simulink model "P4_Combined_Electric_Vehicle"  (R2023b)
settings: Solver=VariableStepAuto  StartTime=0.0  StopTime=10.0  RelTol=1e-3
undefined symbols (not defined in the file or in its folder): batData, carData, motorData
settings Model: Creator=chris  LastModifiedBy=chris

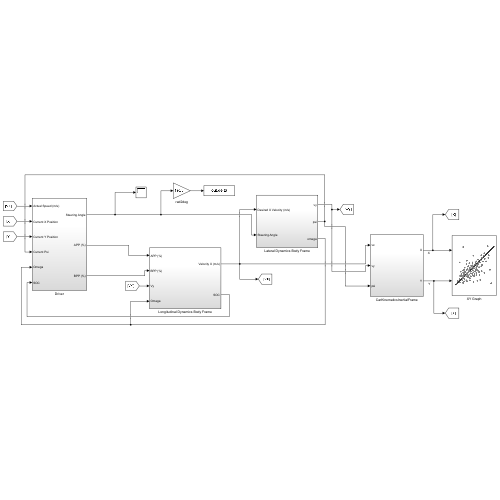
[thumbnail: Simulink's stored preview of the top-level diagram]
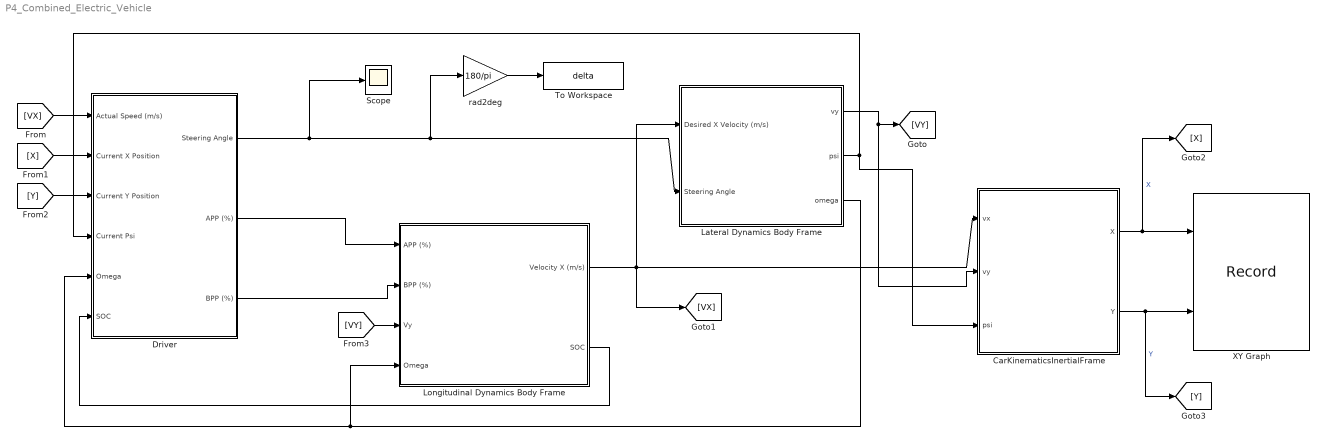
== system P4_Combined_Electric_Vehicle ==
  CarKinematicsInertialFrame : Subsystem
  Driver : Subsystem
  Lateral Dynamics Body Frame : Subsystem
  Longitudinal Dynamics Body Frame : Subsystem
  Scope : Scope
  To Workspace : ToWorkspace  VariableName=delta  SaveFormat=Timeseries  SampleTime=-1
  XY Graph : Record  FileSettingsInternal="{\"entries\":[{\"content\":{\"excelSettings\":{\"content\":{},\"type\":\"Streamout.ExcelSettings\"}},\"type\":\"Streamout.FileSettingStorage\",\"uuid\":\"\"}],\"packageUris\":[\"http:\\/\\/schema.mathworks.com\\/mf0\\/streamout_blocks\\/R2020a\"],\"version\":\"1.0\"}"  Layout=[1 1]  SignalsInternal="{\"entries\":[{\"content\":{\"signals\":[{\"content\":{\"blockPath\":[],\"dimensions\":[1],\"domain\":\"\",\"lineColor\":\"#a2142f\",\"plots\":[1],\"port\":1,\"signalID\":70,\"signalName\":\"XY Graph:1\"},\"type\":\"RecordBlkView.Signal\",\"uuid\":\"\"},{\"content\":{\"blockPath\":[],\"dimensions\":[1],\"domain\":\"\",\"lineColor\":\"#139fff\",\"plots\":[1],\"port\":2,\"signalID\":73,\"signalName\":\"XY Graph:2\"},\"type\":\"RecordBlkView.Signal\",\"uuid\":\"\"}]},\"type\":\"RecordBlkView.InputSignals\",\"uuid\":\"\"}],\"packageUris\":[\"http:\\/\\/schema.mathworks.com\\/mf0\\/streamout_blocks\\/R2020a\"],\"version\":\"1.0\"}"  VisualizationBindings="{\"xyplotplugin\":{\"info\":[{\"series\":[{\"bindingParametersList\":[{\"parameter\":\"X-Axis\",\"signalID\":70,\"signalName\":\"XY Graph:1\"},{\"parameter\":\"Y-Axis\",\"signalID\":73,\"signalName\":\"XY Graph:2\"}],\"seriesID\":10699}],\"subplotID\":1}]}}"  CompatibilityTag=XY
  rad2deg : Gain  Gain=180/pi
  wires:
  [VX] -> Driver/1(Actual Speed (m/s))
  [X] -> Driver/2(Current X Position)
  [Y] -> Driver/3(Current Y Position)
  Driver/2(APP (%)) -> Longitudinal Dynamics Body Frame/1(APP (%))
  Driver/3(BPP (%)) -> Longitudinal Dynamics Body Frame/2(BPP (%))
  [VY] -> Longitudinal Dynamics Body Frame/3(Vy)
  Driver/1(Steering Angle) -> rad2deg/1, Lateral Dynamics Body Frame/2(Steering Angle), Scope/1
  Longitudinal Dynamics Body Frame/1(Velocity X (m/s)) -> Lateral Dynamics Body Frame/1(Desired X Velocity (m/s)), CarKinematicsInertialFrame/1(vx), [VX]
  Longitudinal Dynamics Body Frame/2(SOC) -> Driver/6(SOC)
  rad2deg/1 -> To Workspace/1
  CarKinematicsInertialFrame/1(X) -> XY Graph/1, [X]  "X"
  CarKinematicsInertialFrame/2(Y) -> XY Graph/2, [Y]  "Y"
  Lateral Dynamics Body Frame/1(vy) -> CarKinematicsInertialFrame/2(vy), [VY]
  Lateral Dynamics Body Frame/2(psi) -> CarKinematicsInertialFrame/3(psi), Driver/4(Current Psi)
  Lateral Dynamics Body Frame/3(omega) -> Longitudinal Dynamics Body Frame/4(Omega), Driver/5(Omega)

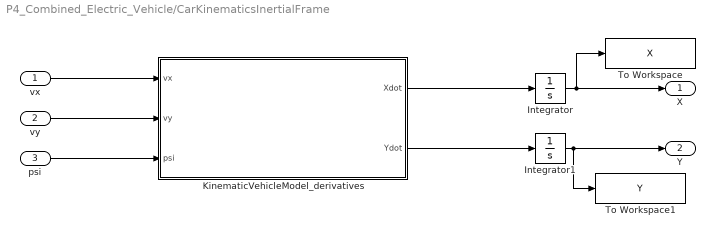
== system P4_Combined_Electric_Vehicle/CarKinematicsInertialFrame ==
  vx : Inport
  vy : Inport  Port=2
  psi : Inport  Port=3
  Integrator : Integrator  InitialCondition=carData.init.X0
  Integrator1 : Integrator  InitialCondition=carData.init.Y0
  KinematicVehicleModel_derivatives : MATLAB Function  TreatAsAtomicUnit=on  mask{obj=carData}
      mask prompts: obj "obj structure"
  To Workspace : ToWorkspace  VariableName=X  SaveFormat=Timeseries  SampleTime=-1
  To Workspace1 : ToWorkspace  VariableName=Y  SaveFormat=Timeseries  SampleTime=-1
  X : Outport
  Y : Outport  Port=2
  wires:
  KinematicVehicleModel_derivatives/1(Xdot) -> Integrator/1
  Integrator/1 -> X/1, To Workspace/1
  psi/1 -> KinematicVehicleModel_derivatives/3(psi)
  Integrator1/1 -> Y/1, To Workspace1/1
  vx/1 -> KinematicVehicleModel_derivatives/1(vx)
  vy/1 -> KinematicVehicleModel_derivatives/2(vy)
  KinematicVehicleModel_derivatives/2(Ydot) -> Integrator1/1

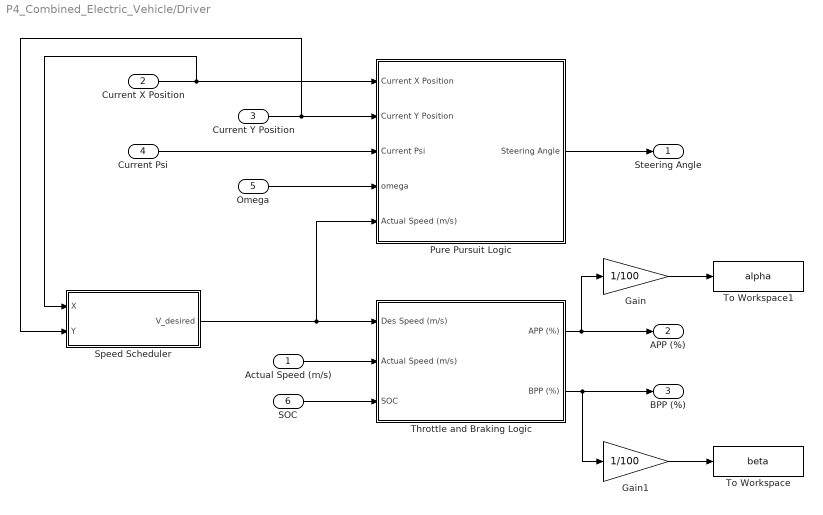
== system P4_Combined_Electric_Vehicle/Driver ==
  Actual Speed (m/s) : Inport
  Current X Position : Inport  Port=2
  Current Y Position : Inport  Port=3
  Current Psi : Inport  Port=4
  Omega : Inport  Port=5
  SOC : Inport  Port=6
  Gain : Gain  Gain=1/100
  Gain1 : Gain  Gain=1/100
  Pure Pursuit Logic : Subsystem
  Speed Scheduler : MATLAB Function  TreatAsAtomicUnit=on
  Throttle and Braking Logic : Subsystem
  To Workspace : ToWorkspace  VariableName=beta  SaveFormat=Timeseries  SampleTime=-1
  To Workspace1 : ToWorkspace  VariableName=alpha  SaveFormat=Timeseries  SampleTime=-1
  Steering Angle : Outport
  APP (%) : Outport  Port=2
  BPP (%) : Outport  Port=3
  wires:
  Actual Speed (m/s)/1 -> Throttle and Braking Logic/2(Actual Speed (m/s))
  SOC/1 -> Throttle and Braking Logic/3(SOC)
  Speed Scheduler/1(V_desired) -> Pure Pursuit Logic/5(Actual Speed (m/s)), Throttle and Braking Logic/1(Des Speed (m/s))
  Omega/1 -> Pure Pursuit Logic/4(omega)
  Current Y Position/1 -> Speed Scheduler/2(Y), Pure Pursuit Logic/2(Current Y Position)
  Current X Position/1 -> Speed Scheduler/1(X), Pure Pursuit Logic/1(Current X Position)
  Current Psi/1 -> Pure Pursuit Logic/3(Current Psi)
  Pure Pursuit Logic/1(Steering Angle) -> Steering Angle/1
  Throttle and Braking Logic/1(APP (%)) -> Gain/1, APP (%)/1
  Throttle and Braking Logic/2(BPP (%)) -> Gain1/1, BPP (%)/1
  Gain1/1 -> To Workspace/1
  Gain/1 -> To Workspace1/1

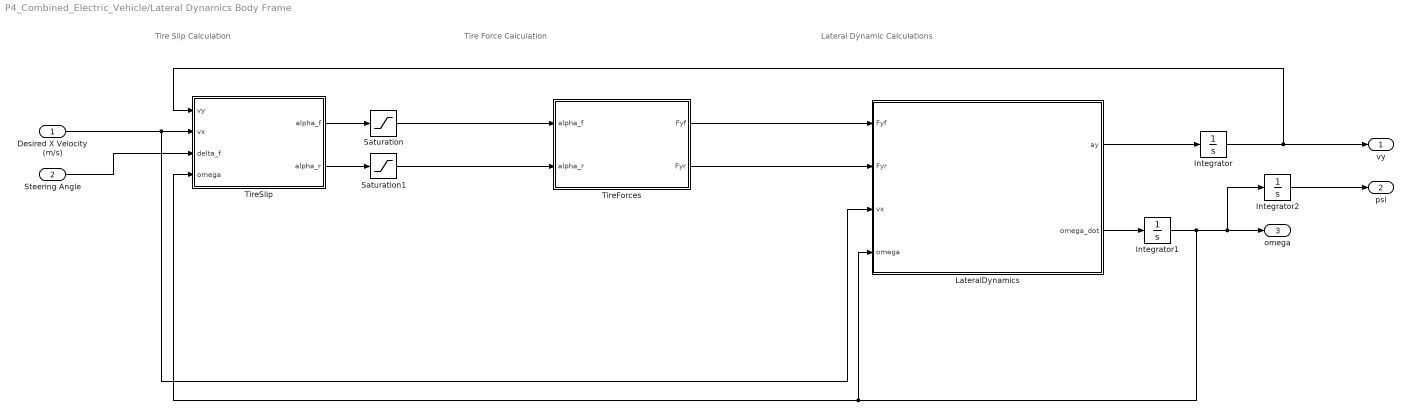
== system P4_Combined_Electric_Vehicle/Lateral Dynamics Body Frame ==
  note: Lateral Dynamic Calculations
  note: Tire Slip Calculation
  note: Tire Force Calculation
  Desired X Velocity (m/s) : Inport
  Steering Angle : Inport  Port=2
  Integrator : Integrator  InitialCondition=carData.init.vy0
  Integrator1 : Integrator  InitialCondition=carData.init.omega0
  Integrator2 : Integrator  InitialCondition=carData.init.psi0
  LateralDynamics : MATLAB Function  TreatAsAtomicUnit=on  mask{obj=carData}
      mask prompts: obj "obj structure"
  Saturation : Saturate  UpperLimit=carData.maxAlpha  LowerLimit=-carData.maxAlpha
  Saturation1 : Saturate  UpperLimit=carData.maxAlpha  LowerLimit=-carData.maxAlpha
  TireForces : MATLAB Function  TreatAsAtomicUnit=on  mask{obj=carData}
      mask prompts: obj "obj structure"
  TireSlip : MATLAB Function  TreatAsAtomicUnit=on  mask{obj=carData}
      mask prompts: obj "obj structure"
  vy : Outport
  psi : Outport  Port=2
  omega : Outport  Port=3
  wires:
  Integrator2/1 -> psi/1
  Steering Angle/1 -> TireSlip/3(delta_f)
  Desired X Velocity (m/s)/1 -> TireSlip/2(vx), LateralDynamics/3(vx)
  Saturation1/1 -> TireForces/2(alpha_r)
  TireForces/2(Fyr) -> LateralDynamics/2(Fyr)
  Saturation/1 -> TireForces/1(alpha_f)
  Integrator1/1 -> Integrator2/1, omega/1, LateralDynamics/4(omega), TireSlip/4(omega)
  Integrator/1 -> vy/1, TireSlip/1(vy)
  TireSlip/2(alpha_r) -> Saturation1/1
  LateralDynamics/2(omega_dot) -> Integrator1/1
  TireForces/1(Fyf) -> LateralDynamics/1(Fyf)
  TireSlip/1(alpha_f) -> Saturation/1
  LateralDynamics/1(ay) -> Integrator/1

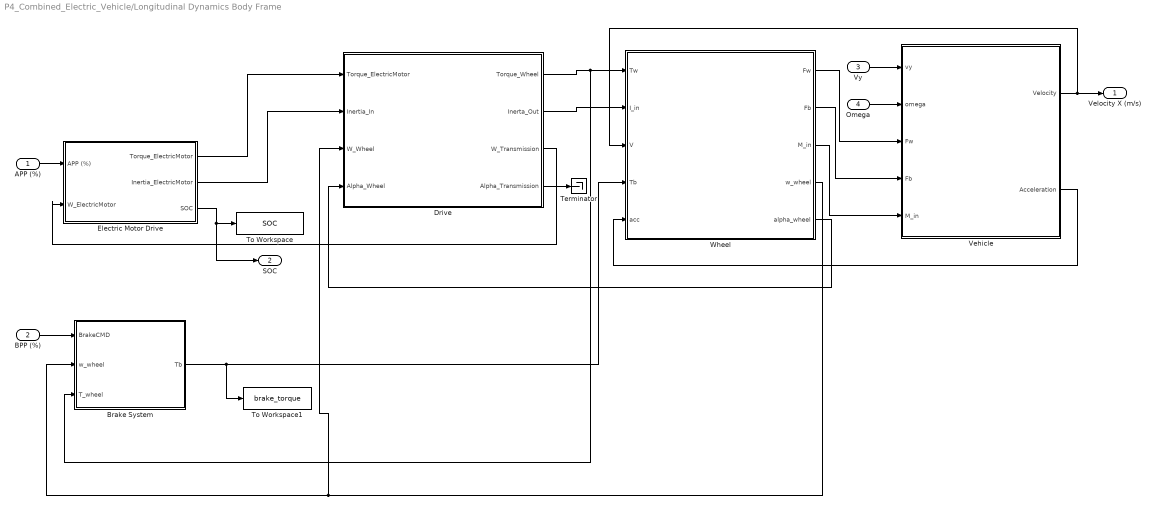
== system P4_Combined_Electric_Vehicle/Longitudinal Dynamics Body Frame ==
  APP (%) : Inport
  BPP (%) : Inport  Port=2
  Vy : Inport  Port=3
  Omega : Inport  Port=4
  Brake System : Subsystem
  Drive : Subsystem
  Electric Motor Drive : Subsystem
  Terminator : Terminator
  To Workspace : ToWorkspace  VariableName=SOC  SaveFormat=Timeseries  SampleTime=-1
  To Workspace1 : ToWorkspace  VariableName=brake_torque  SaveFormat=Timeseries  SampleTime=-1
  Vehicle : Subsystem
  Wheel : Subsystem
  Velocity X (m/s) : Outport
  SOC : Outport  Port=2
  wires:
  Vy/1 -> Vehicle/1(vy)
  Omega/1 -> Vehicle/2(omega)
  APP (%)/1 -> Electric Motor Drive/1(APP (%))
  Electric Motor Drive/3(SOC) -> To Workspace/1, SOC/1
  BPP (%)/1 -> Brake System/1("BrakeCMD ")
  Drive/4(Alpha_Transmission) -> Terminator/1
  Electric Motor Drive/1(Torque_ElectricMotor) -> Drive/1(Torque_ElectricMotor)
  Electric Motor Drive/2(Inertia_ElectricMotor) -> Drive/2(Inertia_In)
  Wheel/3(M_in) -> Vehicle/5("M_in ")
  Wheel/2(Fb) -> Vehicle/4(Fb)
  Wheel/1(Fw) -> Vehicle/3("Fw ")
  Vehicle/2(Acceleration) -> Wheel/5(acc)
  Vehicle/1("Velocity ") -> Wheel/3(V), Velocity X (m/s)/1
  Drive/1(Torque_Wheel) -> Wheel/1(Tw), Brake System/3(T_wheel)
  Drive/2(Inerta_Out) -> Wheel/2(I_in)
  Brake System/1(Tb) -> To Workspace1/1, Wheel/4(Tb)
  Drive/3(W_Transmission) -> Electric Motor Drive/2(W_ElectricMotor)
  Wheel/5(alpha_wheel) -> Drive/4(Alpha_Wheel)
  Wheel/4(w_wheel) -> Drive/3(W_Wheel), Brake System/2("w_wheel ")

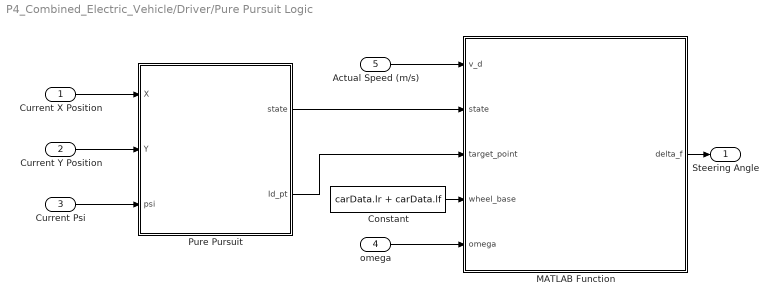
== system P4_Combined_Electric_Vehicle/Driver/Pure Pursuit Logic ==
  Current X Position : Inport
  Current Y Position : Inport  Port=2
  Current Psi : Inport  Port=3
  omega : Inport  Port=4
  Actual Speed (m/s) : Inport  Port=5
  Constant : Constant  Value=carData.lr + carData.lf
  MATLAB Function : MATLAB Function  TreatAsAtomicUnit=on
  Pure Pursuit : MATLAB Function  TreatAsAtomicUnit=on
  Steering Angle : Outport
  wires:
  Current X Position/1 -> Pure Pursuit/1(X)
  Current Y Position/1 -> Pure Pursuit/2(Y)
  Current Psi/1 -> Pure Pursuit/3(psi)
  Actual Speed (m/s)/1 -> MATLAB Function/1(v_d)
  Pure Pursuit/1(state) -> MATLAB Function/2(state)
  omega/1 -> MATLAB Function/5(omega)
  Pure Pursuit/2(Id_pt) -> MATLAB Function/3(target_point)
  MATLAB Function/1(delta_f) -> Steering Angle/1
  Constant/1 -> MATLAB Function/4(wheel_base)

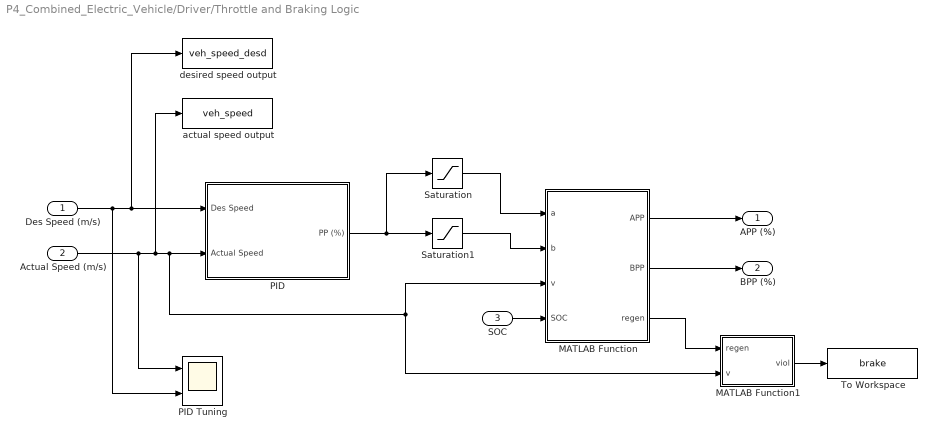
== system P4_Combined_Electric_Vehicle/Driver/Throttle and Braking Logic ==
  Des Speed (m/s) : Inport
  Actual Speed (m/s) : Inport  Port=2
  SOC : Inport  Port=3
  MATLAB Function : MATLAB Function  TreatAsAtomicUnit=on
  MATLAB Function1 : MATLAB Function  TreatAsAtomicUnit=on
  PID : Subsystem
  PID Tuning : Scope  NumInputPorts=2
  Saturation : Saturate  UpperLimit=1  LowerLimit=0
  Saturation1 : Saturate  UpperLimit=0  LowerLimit=-1
  To Workspace : ToWorkspace  VariableName=brake  SaveFormat=Timeseries  SampleTime=-1
  actual speed output : ToWorkspace  VariableName=veh_speed  SaveFormat=Timeseries  SampleTime=-1
  desired speed output : ToWorkspace  VariableName=veh_speed_desd  SaveFormat=Timeseries  SampleTime=-1
  APP (%) : Outport
  BPP (%) : Outport  Port=2
  wires:
  Des Speed (m/s)/1 -> desired speed output/1, PID/1(Des Speed), PID Tuning/2
  Actual Speed (m/s)/1 -> PID Tuning/1, actual speed output/1, MATLAB Function1/2(v), MATLAB Function/3(v), PID/2(Actual Speed)
  SOC/1 -> MATLAB Function/4(SOC)
  MATLAB Function/1(APP) -> APP (%)/1
  MATLAB Function/2(BPP) -> BPP (%)/1
  PID/1(PP (%)) -> Saturation1/1, Saturation/1
  Saturation1/1 -> MATLAB Function/2(b)
  Saturation/1 -> MATLAB Function/1(a)
  MATLAB Function/3(regen) -> MATLAB Function1/1(regen)
  MATLAB Function1/1(viol) -> To Workspace/1

== system P4_Combined_Electric_Vehicle/Longitudinal Dynamics Body Frame/Brake System ==
  "BrakeCMD " : Inport
  "w_wheel " : Inport  Port=2
  T_wheel : Inport  Port=3
  Gain1 : Gain  Gain=10000
  MATLAB Function : MATLAB Function  TreatAsAtomicUnit=on
  Tb : Outport  VectorParamsAs1DForOutWhenUnconnected=off
  wires:
  "BrakeCMD "/1 -> Gain1/1
  T_wheel/1 -> MATLAB Function/3(T_wheel)
  "w_wheel "/1 -> MATLAB Function/2(v)
  Gain1/1 -> MATLAB Function/1(Tbcap)
  MATLAB Function/1(Tb) -> Tb/1

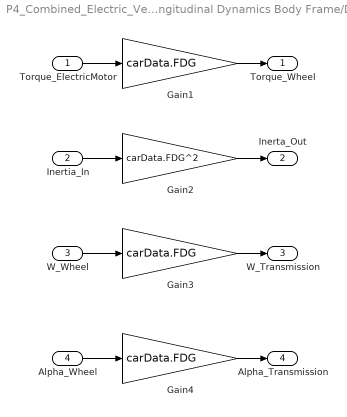
== system P4_Combined_Electric_Vehicle/Longitudinal Dynamics Body Frame/Drive ==
  Torque_ElectricMotor : Inport
  Inertia_In : Inport  Port=2
  W_Wheel : Inport  Port=3
  Alpha_Wheel : Inport  Port=4
  Gain1 : Gain  Gain=carData.FDG
  Gain2 : Gain  Gain=carData.FDG^2
  Gain3 : Gain  Gain=carData.FDG
  Gain4 : Gain  Gain=carData.FDG
  Torque_Wheel : Outport
  Inerta_Out : Outport  Port=2
  W_Transmission : Outport  Port=3
  Alpha_Transmission : Outport  Port=4
  wires:
  Inertia_In/1 -> Gain2/1
  Torque_ElectricMotor/1 -> Gain1/1
  Gain4/1 -> Alpha_Transmission/1
  Gain2/1 -> Inerta_Out/1
  Gain1/1 -> Torque_Wheel/1
  W_Wheel/1 -> Gain3/1
  Gain3/1 -> W_Transmission/1
  Alpha_Wheel/1 -> Gain4/1

== system P4_Combined_Electric_Vehicle/Longitudinal Dynamics Body Frame/Electric Motor Drive ==
  APP (%) : Inport
  W_ElectricMotor : Inport  Port=2
  Battery : Subsystem
  Electric Motor : Subsystem
  Torque_ElectricMotor : Outport
  Inertia_ElectricMotor : Outport  Port=2
  SOC : Outport  Port=3
  wires:
  Electric Motor/3(Inertia_ElectricMotor) -> Inertia_ElectricMotor/1
  Electric Motor/2(Torque_ElectricMotor) -> Torque_ElectricMotor/1
  Battery/2(SOC) -> SOC/1
  Electric Motor/1(I_bat) -> Battery/1(I_battery)
  APP (%)/1 -> Electric Motor/2(APP (%))
  W_ElectricMotor/1 -> Electric Motor/3(W_ElectricMotor)
  Battery/1(V_bat) -> Electric Motor/1(Bat Voltage)

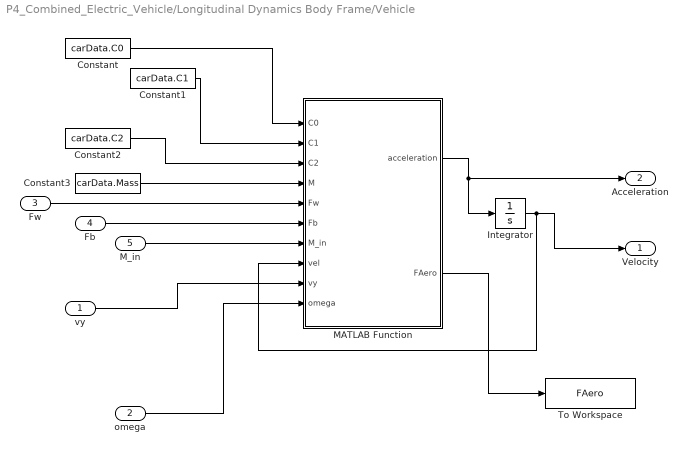
== system P4_Combined_Electric_Vehicle/Longitudinal Dynamics Body Frame/Vehicle ==
  vy : Inport
  omega : Inport  Port=2
  "Fw " : Inport  Port=3
  Fb : Inport  Port=4
  "M_in " : Inport  Port=5
  Constant : Constant  Value=carData.C0
  Constant1 : Constant  Value=carData.C1
  Constant2 : Constant  Value=carData.C2
  Constant3 : Constant  Value=carData.Mass
  Integrator : Integrator  LimitOutput=on  LowerSaturationLimit=0
  MATLAB Function : MATLAB Function  TreatAsAtomicUnit=on
  To Workspace : ToWorkspace  VariableName=FAero  SaveFormat=Timeseries  SampleTime=-1
  "Velocity " : Outport  VectorParamsAs1DForOutWhenUnconnected=off
  Acceleration : Outport  Port=2
  wires:
  "M_in "/1 -> MATLAB Function/7(M_in)
  Constant3/1 -> MATLAB Function/4(M)
  "Fw "/1 -> MATLAB Function/5(Fw)
  Constant/1 -> MATLAB Function/1(C0)
  Constant2/1 -> MATLAB Function/3(C2)
  Fb/1 -> MATLAB Function/6(Fb)
  Integrator/1 -> "Velocity "/1, MATLAB Function/8(vel)
  MATLAB Function/1(acceleration) -> Integrator/1, Acceleration/1
  Constant1/1 -> MATLAB Function/2(C1)
  vy/1 -> MATLAB Function/9(vy)
  omega/1 -> MATLAB Function/10(omega)
  MATLAB Function/2(FAero) -> To Workspace/1

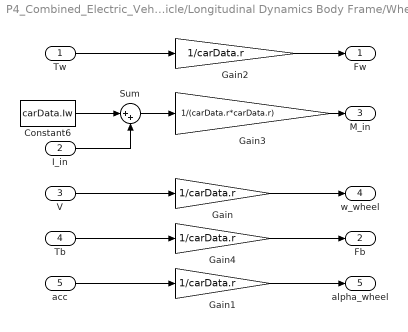
== system P4_Combined_Electric_Vehicle/Longitudinal Dynamics Body Frame/Wheel ==
  Tw : Inport
  I_in : Inport  Port=2
  V : Inport  Port=3
  Tb : Inport  Port=4
  acc : Inport  Port=5
  Constant6 : Constant  Value=carData.Iw
  Gain{,1..2,4} (4 alike) : Gain  Gain=1/carData.r
  Gain3 : Gain  Gain=1/(carData.r*carData.r)
  Sum : Sum  Inputs=|++
  Fw : Outport
  Fb : Outport  Port=2
  M_in : Outport  Port=3
  w_wheel : Outport  Port=4
  alpha_wheel : Outport  Port=5
  wires:
  acc/1 -> Gain1/1
  Gain1/1 -> alpha_wheel/1
  Constant6/1 -> Sum/1
  Gain3/1 -> M_in/1
  Sum/1 -> Gain3/1
  Gain4/1 -> Fb/1
  I_in/1 -> Sum/2
  V/1 -> Gain/1
  Tw/1 -> Gain2/1
  Gain/1 -> w_wheel/1
  Gain2/1 -> Fw/1
  Tb/1 -> Gain4/1

== system P4_Combined_Electric_Vehicle/Driver/Throttle and Braking Logic/PID ==
  Des Speed : Inport
  Actual Speed : Inport  Port=2
  PP (%) : Outport
  wires:
  Des Speed/1 -> PP (%)/1

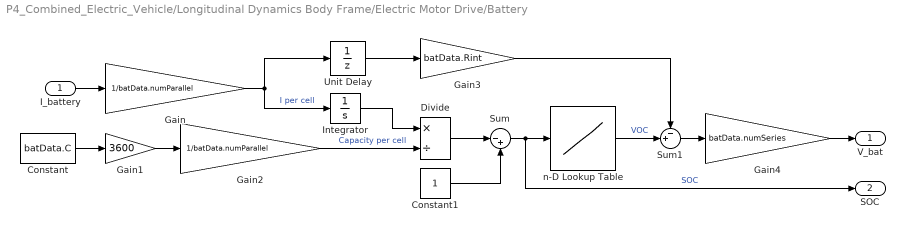
== system P4_Combined_Electric_Vehicle/Longitudinal Dynamics Body Frame/Electric Motor Drive/Battery ==
  I_battery : Inport
  Constant : Constant  Value=batData.C
  Constant1 : Constant
  Divide : Product  Inputs=*/
  Gain : Gain  Gain=1/batData.numParallel
  Gain1 : Gain  Gain=3600
  Gain2 : Gain  Gain=1/batData.numParallel
  Gain3 : Gain  Gain=batData.Rint
  Gain4 : Gain  Gain=batData.numSeries
  Integrator : Integrator
  Sum : Sum  Inputs=|-+
  Sum1 : Sum  Inputs=-+|
  Unit Delay : UnitDelay  SampleTime=-1  HasFrameUpgradeWarning=on
  n-D Lookup Table : Lookup_n-D  NumberOfTableDimensions=1  BreakpointsForDimension1=batData.SOC  BreakpointsForDimension3=[5, 7]  Table=batData.OCV  InternalRulePriority=Speed  RndMeth=Simplest
  V_bat : Outport
  SOC : Outport  Port=2
  wires:
  I_battery/1 -> Gain/1
  Gain/1 -> Unit Delay/1, Integrator/1  "I per cell"
  Constant/1 -> Gain1/1
  Gain1/1 -> Gain2/1
  Gain2/1 -> Divide/2  "Capacity per cell"
  Integrator/1 -> Divide/1
  Divide/1 -> Sum/1
  Constant1/1 -> Sum/2
  Sum/1 -> SOC/1, n-D Lookup Table/1  "SOC"
  Unit Delay/1 -> Gain3/1
  n-D Lookup Table/1 -> Sum1/2  "VOC"
  Gain3/1 -> Sum1/1
  Gain4/1 -> V_bat/1
  Sum1/1 -> Gain4/1

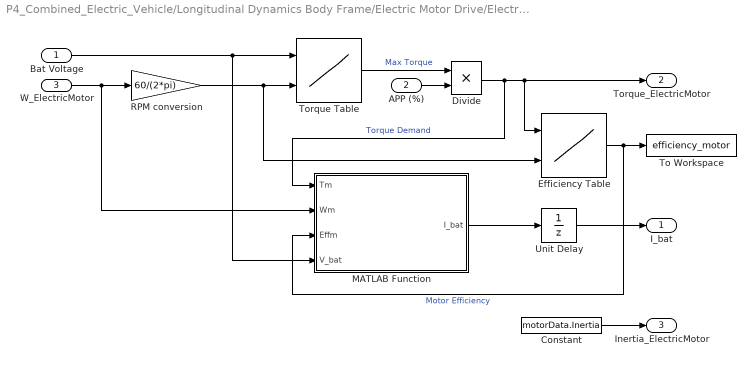
== system P4_Combined_Electric_Vehicle/Longitudinal Dynamics Body Frame/Electric Motor Drive/Electric Motor ==
  Bat Voltage : Inport
  APP (%) : Inport  Port=2
  W_ElectricMotor : Inport  Port=3
  Constant : Constant  Value=motorData.Inertia
  Divide : Product  Inputs=**
  Efficiency Table : Lookup_n-D  BreakpointsForDimension1=motorData.eta_torque  BreakpointsForDimension2=motorData.eta_speed  BreakpointsForDimension3=[5, 7]  Table=motorData.eta_val  ExtrapMethod=Clip  UseLastTableValue=on  InternalRulePriority=Speed  RndMeth=Simplest
      settings: InputPortMap=u0,u1
  MATLAB Function : MATLAB Function  TreatAsAtomicUnit=on
  RPM conversion : Gain  Gain=60/(2*pi)
  To Workspace : ToWorkspace  VariableName=efficiency_motor  SaveFormat=Timeseries  SampleTime=-1
  Torque Table : Lookup_n-D  BreakpointsForDimension1=motorData.vbus  BreakpointsForDimension2=motorData.rpm  BreakpointsForDimension3=[5, 7]  Table=motorData.maxtorque  ExtrapMethod=Clip  UseLastTableValue=on  InternalRulePriority=Speed  RndMeth=Simplest
      settings: InputPortMap=u0,u1
  Unit Delay : UnitDelay  SampleTime=-1  HasFrameUpgradeWarning=on
  I_bat : Outport
  Torque_ElectricMotor : Outport  Port=2
  Inertia_ElectricMotor : Outport  Port=3
  wires:
  W_ElectricMotor/1 -> MATLAB Function/2(Wm), RPM conversion/1
  Bat Voltage/1 -> MATLAB Function/4(V_bat), Torque Table/1
  RPM conversion/1 -> Efficiency Table/2, Torque Table/2
  Torque Table/1 -> Divide/1  "Max Torque"
  APP (%)/1 -> Divide/2
  Divide/1 -> MATLAB Function/1(Tm), Torque_ElectricMotor/1, Efficiency Table/1  "Torque Demand"
  Efficiency Table/1 -> MATLAB Function/3(Effm), To Workspace/1  "Motor Efficiency"
  Constant/1 -> Inertia_ElectricMotor/1
  MATLAB Function/1(I_bat) -> Unit Delay/1
  Unit Delay/1 -> I_bat/1

== matlab function P4_Combined_Electric_Vehicle/Lateral Dynamics Body Frame/LateralDynamics ==
  data: Fyf input; Fyr input size=1; vx input; omega input; ay output; obj parameter; omega_dot output
function [ay, omega_dot] = fcn(Fyf, Fyr, vx, omega, obj)

Fy = Fyf + Fyr;
ay = Fy / obj.Mass - omega * vx;
        
M  = Fyf * obj.lf - Fyr * obj.lr;        
omega_dot = M / obj.Inertia;        

end

== matlab function P4_Combined_Electric_Vehicle/Lateral Dynamics Body Frame/TireForces ==
  data: alpha_f input; alpha_r input; Fyf output; obj parameter; Fyr output
function [Fyf, Fyr] = fcn(alpha_f, alpha_r, obj)

Fyf = min(obj.Fyfmax,obj.Calpha_f * alpha_f);
Fyr = min(obj.Fyrmax, obj.Calpha_r * alpha_r);
end

== matlab function P4_Combined_Electric_Vehicle/Lateral Dynamics Body Frame/TireSlip ==
  data: vy input size=1; vx input; delta_f input size=1; omega input; alpha_f output; obj parameter; alpha_r output
function [alpha_f, alpha_r] = fcn(vy,  vx, delta_f, omega, obj)


if abs(vx)> obj.vx_threshold1
      alpha_f = delta_f - (vy + omega * obj.lf) / vx;
      alpha_r = - (vy - omega * obj.lr) / vx;
else
      alpha_f = 0;
      alpha_r = 0;
end



end

== matlab function P4_Combined_Electric_Vehicle/Driver/Throttle and Braking Logic/MATLAB Function ==
  data: a input; b input; v input; APP output; BPP output; SOC input; regen output
function [APP,BPP, regen] = fcn(a, b, v, SOC)

if v < 5
    regen = 0;
elseif 5 <= v && v < 25
    regen = b*(1-0.05);
end

== matlab function P4_Combined_Electric_Vehicle/Driver/Speed Scheduler ==
  data: X input; V_desired output; Y input
function V_desired = fcn(X, Y)

V_desired = X + Y;

== matlab function P4_Combined_Electric_Vehicle/Driver/Throttle and Braking Logic/MATLAB Function1 ==
  data: regen input; viol output; v input
function viol = violfcn(regen, v)
    speed = (3600/1600)*v;
    if speed < 5
        regen_vio = 0;
        if regen == regen_vio
            viol = 0;
        else
            viol = 1;
        end

    elseif speed == 25
        regen_vio = 0.95;
        if regen == regen_vio
            viol = 0;
        else
            viol = 1;
        end

    elseif v > 25
        regen_vio = 0.95;
        if regen == regen_vio
            viol = 0;
        else
            viol = 1;
        end
    else
        regen_vio = ((0.95/20)*speed) - 0.2375;
        if regen == regen_vio
            viol = 0;
        else
            viol = 1;
        end
    end

== matlab function P4_Combined_Electric_Vehicle/Driver/Pure Pursuit Logic/Pure Pursuit ==
  data: state output; X input; Y input; psi input; Id_pt output
function [state, Id_pt]= fcn(X, Y, psi)

y = u;

== matlab function P4_Combined_Electric_Vehicle/Driver/Pure Pursuit Logic/MATLAB Function ==
  data: v_d input; state input; delta_f output; target_point input; wheel_base input; omega input
function delta_f = fcn(v_d, state, target_point, wheel_base, omega)

y = u;

== matlab function P4_Combined_Electric_Vehicle/CarKinematicsInertialFrame/KinematicVehicleModel_derivatives ==
  data: vx input; vy input; psi input size=1; Xdot output; Ydot output
function [Xdot, Ydot] = fcn(vx, vy, psi)
    temp = TF(psi) * [vx;vy]; 
    Xdot = temp(1);
    Ydot = temp(2);
  
end

function y = TF(psi)
    y = [cos(psi), -sin(psi); sin(psi), cos(psi)];
end

== matlab function P4_Combined_Electric_Vehicle/Longitudinal Dynamics Body Frame/Electric Motor Drive/Electric Motor/MATLAB Function ==
  data: Tm input; I_bat output; Wm input; Effm input; V_bat input
function I_bat = fcn(Tm, Wm, Effm, V_bat)
Pm = Tm * Wm;
Sgn_Pm = Pm / (abs(Pm) + 0.001);
I_bat = ( Pm * (Effm^Sgn_Pm) ) / V_bat;

== matlab function P4_Combined_Electric_Vehicle/Longitudinal Dynamics Body Frame/Brake System/MATLAB Function ==
  data: Tbcap input; Tb output; v input; T_wheel input
function Tb = fcn(Tbcap,v, T_wheel)

if Tbcap == 0
    Tb = -T_wheel;
else
    Tb = -(Tbcap * (v/(abs(v)+0.001)));

end
%Tb = Tbcap;
% GO TO LONGITUDINAL Dynamics SLIDES(slide 13) AND ADD THE INFORMATION HERE:
% friction on pad =1, geometric = 1
% brake in locked / un-locked state
% torque = applied torque coming from wheels (for locked),
% Alpha_value(brakepercent)X gain(np_max:10000)x sin approximation of the
% angular velocity of the wheel (continuation)
% torque =  uses friction on the pad alpha_value(brakepercent)X gain(np_max:10000)

% LOCKED-STATE






% UNLOCKED-STATE

== matlab function P4_Combined_Electric_Vehicle/Longitudinal Dynamics Body Frame/Vehicle/MATLAB Function ==
  data: C0 input; acceleration output; C1 input; C2 input; M input; Fw input; Fb input; M_in input; vel input; vy input; omega input; FAero output
function [acceleration, FAero]   = vehicle(C0,C1,C2,M,Fw,Fb,M_in,vel,vy,omega)

FAero = C0 + C1*vel + C2*(vel)^2;
acceleration = ((Fw-Fb)-FAero)/(M+M_in)+vy*omega;

end
